simulink subsystem "body_dyn_and_kin"  (R2024a)
settings: Solver=VariableStepAuto  StartTime=0.0  StopTime=10.0  RelTol=1e-3
libraries: aerolibutil x2, matrix_library x1, sharedutil x1
settings Model: Creator=joshu  LastModifiedBy=joshu

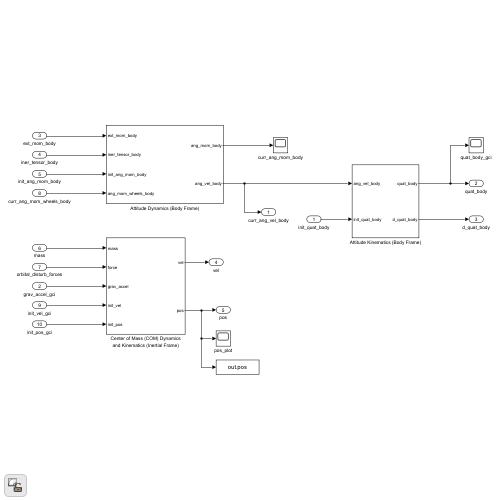
[thumbnail: Simulink's stored preview of the top-level diagram]
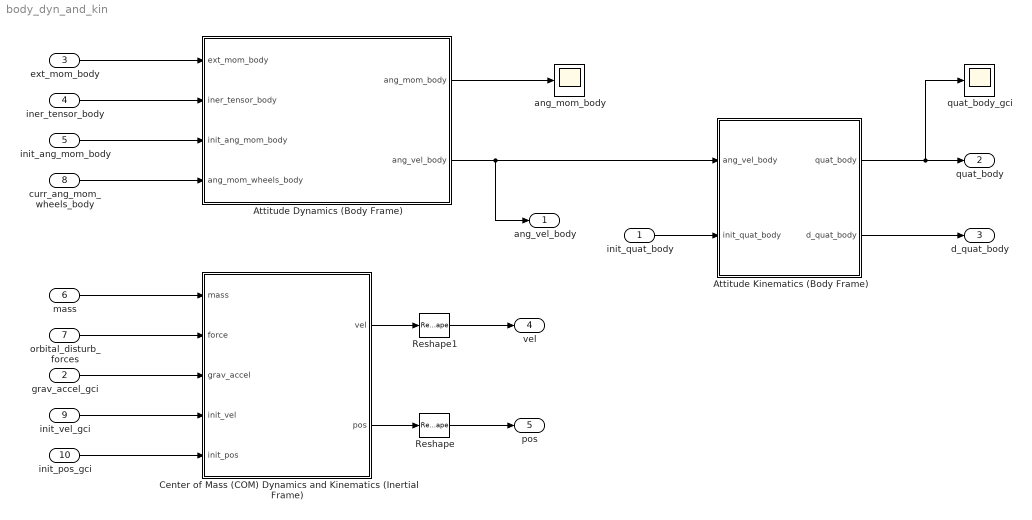
== system body_dyn_and_kin ==
  init_quat_body : Inport
  grav_accel_gci : Inport  Port=2
  ext_mom_body : Inport  Port=3
  iner_tensor_body : Inport  Port=4
  init_ang_mom_body : Inport  Port=5
  mass : Inport  Port=6
  orbital_disturb_forces : Inport  Port=7
  curr_ang_mom_wheels_body : Inport  Port=8
  init_vel_gci : Inport  Port=9
  init_pos_gci : Inport  Port=10
  Attitude Dynamics (Body Frame) : Subsystem
  Attitude Kinematics (Body Frame) : Subsystem
  Center of Mass (COM) Dynamics and Kinematics (Inertial Frame) : Subsystem
  Reshape : Reshape
  Reshape1 : Reshape
  ang_mom_body : Scope
  quat_body_gci : Scope
  ang_vel_body : Outport
  quat_body : Outport  Port=2
  d_quat_body : Outport  Port=3
  vel : Outport  Port=4
  pos : Outport  Port=5
  wires:
  init_quat_body/1 -> Attitude Kinematics (Body Frame)/2(init_quat_body)
  grav_accel_gci/1 -> Center of Mass (COM) Dynamics and Kinematics (Inertial Frame)/3(grav_accel)
  ext_mom_body/1 -> Attitude Dynamics (Body Frame)/1(ext_mom_body)
  Attitude Dynamics (Body Frame)/2(ang_vel_body) -> Attitude Kinematics (Body Frame)/1(ang_vel_body), ang_vel_body/1
  iner_tensor_body/1 -> Attitude Dynamics (Body Frame)/2(iner_tensor_body)
  init_vel_gci/1 -> Center of Mass (COM) Dynamics and Kinematics (Inertial Frame)/4(init_vel)
  orbital_disturb_forces/1 -> Center of Mass (COM) Dynamics and Kinematics (Inertial Frame)/2(force)
  curr_ang_mom_wheels_body/1 -> Attitude Dynamics (Body Frame)/4(ang_mom_wheels_body)
  init_pos_gci/1 -> Center of Mass (COM) Dynamics and Kinematics (Inertial Frame)/5(init_pos)
  Center of Mass (COM) Dynamics and Kinematics (Inertial Frame)/2(pos) -> Reshape/1
  Attitude Kinematics (Body Frame)/2(d_quat_body) -> d_quat_body/1
  Attitude Kinematics (Body Frame)/1(quat_body) -> quat_body/1, quat_body_gci/1
  mass/1 -> Center of Mass (COM) Dynamics and Kinematics (Inertial Frame)/1(mass)
  init_ang_mom_body/1 -> Attitude Dynamics (Body Frame)/3(init_ang_mom_body)
  Attitude Dynamics (Body Frame)/1(ang_mom_body) -> ang_mom_body/1
  Center of Mass (COM) Dynamics and Kinematics (Inertial Frame)/1(vel) -> Reshape1/1
  Reshape/1 -> pos/1
  Reshape1/1 -> vel/1

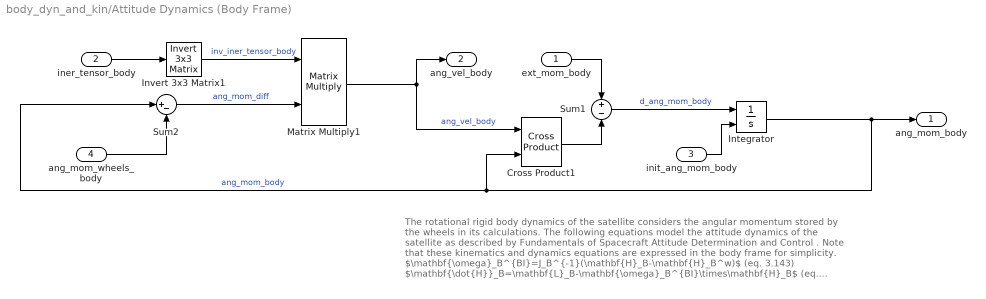
== system body_dyn_and_kin/Attitude Dynamics (Body Frame) ==
  note: The rotational rigid body dynamics of the satellite considers the angular momentum stored by the wheels in its calculations. The following equations model the attitude dynamics of the satellite as described by Fundamentals of Spacecraft Attitude Determination and Control . Note that these kinematics and dynamics equations are expressed in the body frame for simplicity.
      |
      | $\mathbf{\omega}_B^{BI}=J_B^{-1}(\mathbf{H}_B-\mathbf{H}_B^w)$ (eq. 3.143)
      | $\mathbf{\dot{H}}_B=\mathbf{L}_B-\mathbf{\omega}_B^{BI}\times\mathbf{H}_B$ (eq. 3.80)
      |
      | $\mathbf{\omega}_B^{BI}$ - angular velocity of satellite in body frame
      | $J_B$ - inertia tensor of satellite in body frame
      | $\mathbf{H}_B$ - total angular momentum of satellite in body frame
      | $\mathbf{H}_B^w$ - total angular momentum of wheels in body frame
      | $\mathbf{L}_B$ - moment applied to spacecraft in the body frame
  ext_mom_body : Inport
  iner_tensor_body : Inport  Port=2
  init_ang_mom_body : Inport  Port=3
  ang_mom_wheels_body : Inport  Port=4
  Cross Product1 : matrix_library/Cross Product
  Integrator : Integrator  InitialConditionSource=external
  Invert 3x3 Matrix1 : aerolibutil/Invert  3x3 Matrix
  Matrix Multiply1 : Product  Multiplication=Matrix(*)
  Sum1 : Sum  Inputs=+-
  Sum2 : Sum  Inputs=|+-
  ang_mom_body : Outport
  ang_vel_body : Outport  Port=2
  wires:
  Cross Product1/1 -> Sum1/2
  ext_mom_body/1 -> Sum1/1
  Sum1/1 -> Integrator/1  "d_ang_mom_body"
  Sum2/1 -> Matrix Multiply1/2  "ang_mom_diff"
  Matrix Multiply1/1 -> ang_vel_body/1, Cross Product1/1  "ang_vel_body"
  init_ang_mom_body/1 -> Integrator/2
  Integrator/1 -> Cross Product1/2, Sum2/1, ang_mom_body/1  "ang_mom_body"
  ang_mom_wheels_body/1 -> Sum2/2
  iner_tensor_body/1 -> Invert 3x3 Matrix1/1
  Invert 3x3 Matrix1/1 -> Matrix Multiply1/1  "inv_iner_tensor_body"

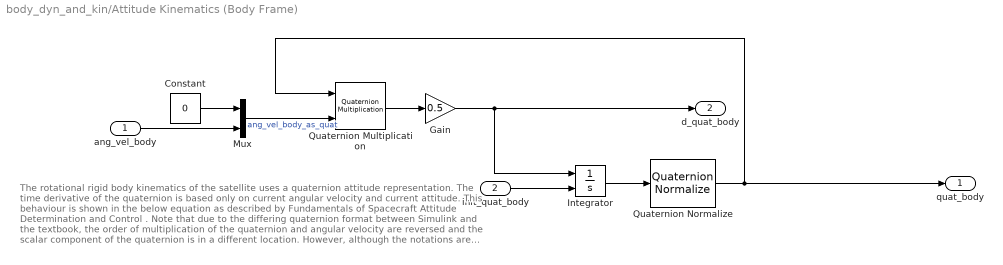
== system body_dyn_and_kin/Attitude Kinematics (Body Frame) ==
  note: The rotational rigid body kinematics of the satellite uses a quaternion attitude representation. The time derivative of the quaternion is based only on current angular velocity and current attitude. This behaviour is shown in the below equation as described by Fundamentals of Spacecraft Attitude Determination and Control . Note that due to the differing quaternion format between Simulink and the textbook, the order of multiplication of the quaternion and angular velocity are reversed and the scalar component of the quaternion is in a different location. However, although the notations are different, they are functionally the same.
      |
      | $\mathbf{\dot{q}}_{BI}=\frac{1}{2}\mathbf{q}_{BI}\cdot\mathbf{\omega}_B^{BI}=\frac{1}{2}\mathbf{q}_{BI}\cdot\left[\matrix{0 \cr \mathbf{\omega}_B^{BI}}\right]$ (eq. 3.79d)
      |
      | Note that in the above equation, multiplication between a quaternion and vector requires transforming the vector to a quaternion with scalar component of 0, as seen on the RHS.
      |
      | $\mathbf{q}_{BI}$ - current attitude of the spacecraft (rotation from inertial frame to body frame as specified in the inertial frame)
      | $\mathbf{\omega}_{B}^{BI}$ - angular velocity of satellite in body frame
  ang_vel_body : Inport
  init_quat_body : Inport  Port=2
  Constant : Constant  Value=0
  Gain : Gain  Gain=0.5
  Integrator : Integrator  InitialConditionSource=external
  Mux : Mux  Inputs=2
  Quaternion Multiplication : aerolibutil/Quaternion Multiplication
  Quaternion Normalize : sharedutil/Quaternion Normalize  aMode=aMode
  quat_body : Outport  PortDimensions=4
  d_quat_body : Outport  Port=2  PortDimensions=4
  wires:
  init_quat_body/1 -> Integrator/2
  Quaternion Normalize/1 -> Quaternion Multiplication/1, quat_body/1
  Gain/1 -> Integrator/1, d_quat_body/1
  Integrator/1 -> Quaternion Normalize/1
  Mux/1 -> Quaternion Multiplication/2  "ang_vel_body_as_quat"
  Quaternion Multiplication/1 -> Gain/1
  ang_vel_body/1 -> Mux/2
  Constant/1 -> Mux/1

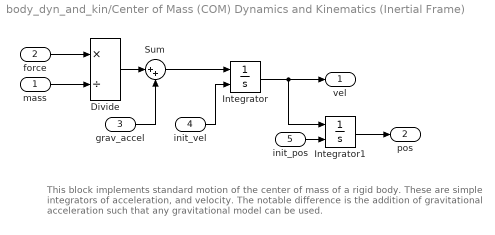
== system body_dyn_and_kin/Center of Mass (COM) Dynamics and Kinematics (Inertial Frame) ==
  note: This block implements standard motion of the center of mass of a rigid body. These are simple integrators of acceleration, and velocity. The notable difference is the addition of gravitational acceleration such that any gravitational model can be used.
  mass : Inport
  force : Inport  Port=2
  grav_accel : Inport  Port=3
  init_vel : Inport  Port=4
  init_pos : Inport  Port=5
  Divide : Product  Inputs=*/
  Integrator : Integrator  InitialConditionSource=external
  Integrator1 : Integrator  InitialConditionSource=external
  Sum : Sum  Inputs=|++
  vel : Outport
  pos : Outport  Port=2
  wires:
  Sum/1 -> Integrator/1
  Integrator1/1 -> pos/1
  Integrator/1 -> Integrator1/1, vel/1
  force/1 -> Divide/1
  mass/1 -> Divide/2
  grav_accel/1 -> Sum/2
  Divide/1 -> Sum/1
  init_pos/1 -> Integrator1/2
  init_vel/1 -> Integrator/2
